simulink model "ContinuosBuck_Offine_Control4"  (R2025a)
settings: Solver=VariableStepAuto  StartTime=0.0  StopTime=SimTime  RelTol=RelativeTolerance
undefined symbols (not defined in the file): C_buck, Iout_buck, kd, ki, kp, L_buck, R, Tsim, Vg, Vout_buck
libraries: slpidlib x1, spsPWMGeneratorDCDCLib x1
settings Model: Creator=Andres  LastModifiedBy=Andres
settings DataIOCC: ReturnWorkspaceOutputs=off  SignalLoggingName=ResultCont

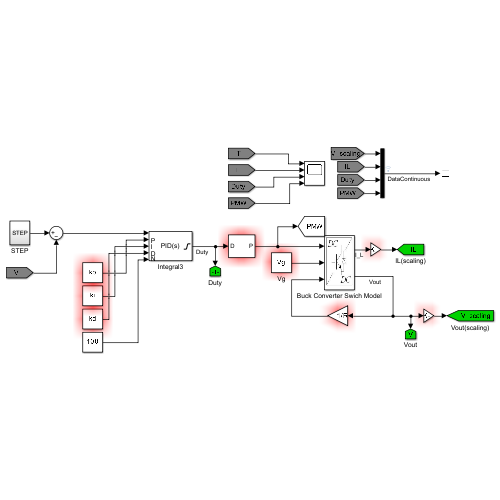
[thumbnail: Simulink's stored preview of the top-level diagram]
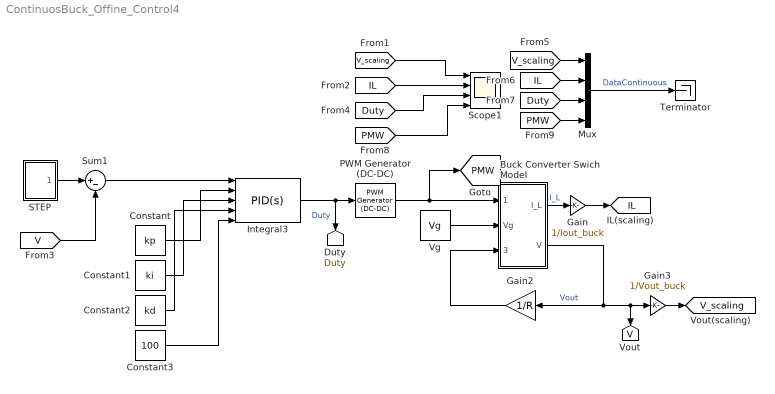
== system ContinuosBuck_Offine_Control4 ==
  Buck Converter Swich Model : Subsystem
      mask Display: image('$imagefile'); % Use "Edit Image" on toolstrip to change.
  Constant : Constant  Value=kp
  Constant1 : Constant  Value=ki
  Constant2 : Constant  Value=kd
  Constant3 : Constant  Value=100
  Gain : Gain  Gain=1/Iout_buck
  Gain2 : Gain  Gain=1/R
  Gain3 : Gain  Gain=1/Vout_buck
  Integral3 : slpidlib/PID Controller  Controller=PID  Form=Parallel  TimeDomain=Continuous-time  UseExternalTs=on  SampleTime=-1  IntegratorMethod=Trapezoidal  FilterMethod=Forward Euler  ControllerParametersSource=external  P=0  I=63.9226  UseKiTs=off  D=0  UseExternalDerivativeSource=off  N=100  UseFilter=on  TunerSelectOption=Transfer Function Based (PID Tuner App)  InitialConditionSource=internal  InitialConditionForIntegrator=0  InitialConditionForFilter=0  DifferentiatorICPrevScaledInput=0  ExternalReset=none  IgnoreLimit=on  TrackingMode=off  Kt=1  LimitOutput=on  SatLimitsSource=internal  UpperSaturationLimit=0.98  LowerSaturationLimit=0  LinearizeAsGain=on  AntiWindupMode=clamping  Kb=1  LimitIntegrator=off  UpperIntegratorSaturationLimit=inf  LowerIntegratorSaturationLimit=-inf  POutMin=[]  POutMax=[]  IOutMin=[]  IOutMax=[]  DOutMin=[]  DOutMax=[]  NOutMin=[]  NOutMax=[]  SumOutMin=[]  SumOutMax=[]  SaturationOutMin=[]  SaturationOutMax=[]  PParamMin=[]  PParamMax=[]  IParamMin=[]  IParamMax=[]  DParamMin=[]  DParamMax=[]  NParamMin=[]  NParamMax=[]  KbParamMin=[]  KbParamMax=[]  KtParamMin=[]  KtParamMax=[]  KbOutMin=[]  KbOutMax=[]  KtOutMin=[]  KtOutMax=[]  IntegratorOutMin=[]  IntegratorOutMax=[]  FilterOutMin=[]  FilterOutMax=[]  SumI1OutMin=[]  SumI1OutMax=[]  SumI2OutMin=[]  SumI2OutMax=[]  SumI3OutMin=[]  SumI3OutMax=[]  SumI4OutMin=[]  SumI4OutMax=[]  SumDOutMin=[]  SumDOutMax=[]  DifferentiatorOutMin=[]  DifferentiatorOutMax=[]  FilterDiffOutCoefMin=[]  FilterDiffOutCoefMax=[]  ReciprocalOutMin=[]  ReciprocalOutMax=[]  SumDenOutMin=[]  SumDenOutMax=[]  SumNumOutMin=[]  SumNumOutMax=[]  DivideOutMin=[]  DivideOutMax=[]  UdiffTsProdOutMin=[]  UdiffTsProdOutMax=[]  NTsProdOutMin=[]  NTsProdOutMax=[]  UintegralTsProdOutMin=[]  UintegralTsProdOutMax=[]  UngainTsProdOutMin=[]  UngainTsProdOutMax=[]  ClampingZeroOutDataTypeStr=Inherit: Inherit via back propagation  ClampingZeroOutMin=[]  ClampingZeroOutMax=[]  FilterDenConstantOutDataTypeStr=Inherit: Inherit via back propagation  FilterDenConstantOutMin=[]  FilterDenConstantOutMax=[]  PCopyOutDataTypeStr=Inherit: Inherit via back propagation  PCopyOutMin=[]  PCopyOutMax=[]  NCopyOutDataTypeStr=Inherit: Inherit via back propagation  NCopyOutMin=[]  NCopyOutMax=[]  IntegratorContinuousStateAttributes=''  IntegratorStateMustResolveToSignalObject=off  IntegratorRTWStateStorageClass=Auto  FilterContinuousStateAttributes=''  FilterStateMustResolveToSignalObject=off  FilterRTWStateStorageClass=Auto  ParallelPVariant=ExternalParameters  IdealPVariant=Disabled  IVariant=ExternalParameters  DVariant=ExternalParameters  IntegratorVariant=Continuous  SatVariant=Enabled  AWVariant=ContClampingParallel  PCopyVariant=Disabled  TRVariant=Disabled  FdbkBlocksVariant=Forward  IdealPFdbkVariant=Disabled  SatFdbkVariant=Disabled  DerivativeFilterVariant=ContFilter  NVariant=ExternalParameters  NCopyVariant=Disabled  FilterICVariant=InternalICsFilter  IntegratorICVariant=InternalICs  ExternalResetVariant=Disabled  TRSumVariant=Passthrough  SumFdbkVariant=Disabled  SumVariant=Sum_PID  TsampFilterVariant=InternalTs  TsampNgainVariant=Passthrough  TsampIntegralVariant=Disabled_SignalSpec  ExternalSaturationOutDataTypeStr=Inherit: Same as second input  DerivativeSourceVariant=ErrorSignal  PreIntVariant=InternalPreInt
  Mux : Mux
  PWM Generator (DC-DC) : spsPWMGeneratorDCDCLib/PWM Generator (DC-DC)  Fsw=f_sw  Ts=0
  STEP : Subsystem
  Scope1 : Scope  NumInputPorts=4
      settings: ActiveDisplayYMinimum=-0.19152108023888853  ActiveDisplayYMaximum=1.7236897221499974  YLabel=Voltage (V)
  Sum1 : Sum  Inputs=|+-
  Terminator : Terminator
  Vg : Constant  Value=Vg  SampleTime=-1
  tag scope: Duty=global, IL=global, PMW=global, V=global, V_scaling=global
  wires:
  Integral3/1 -> [Duty], PWM Generator (DC-DC)/1  "Duty"
  STEP/1(STEP) -> Sum1/1
  [V] -> Sum1/2
  Sum1/1 -> Integral3/1
  Gain2/1 -> Buck Converter Swich Model/3(I_load)
  Buck Converter Swich Model/1(I_L) -> Gain/1  "I_L"
  Buck Converter Swich Model/2(V) -> Gain2/1, [V], Gain3/1  "Vout"
  PWM Generator (DC-DC)/1 -> [PMW], Buck Converter Swich Model/1(PWM)
  Vg/1 -> Buck Converter Swich Model/2(Vg)
  Mux/1 -> Terminator/1  "DataContinuous"
  Gain3/1 -> [V_scaling]
  Gain/1 -> [IL]
  [V_scaling] -> Scope1/1
  [IL] -> Scope1/2
  [Duty] -> Scope1/3
  [V_scaling] -> Mux/1
  [IL] -> Mux/2
  [Duty] -> Mux/3
  [PMW] -> Scope1/4
  [PMW] -> Mux/4
  Constant/1 -> Integral3/2
  Constant1/1 -> Integral3/3
  Constant2/1 -> Integral3/4
  Constant3/1 -> Integral3/5

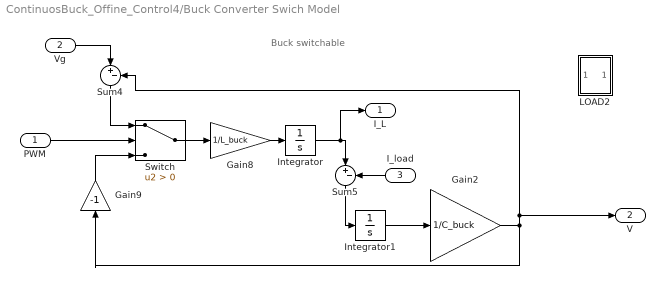
== system ContinuosBuck_Offine_Control4/Buck Converter Swich Model ==
  note: Buck switchable
  PWM : Inport
  Vg : Inport  Port=2
  I_load : Inport  Port=3
  Gain2 : Gain  Gain=1/C_buck
  Gain8 : Gain  Gain=1/L_buck
  Gain9 : Gain  Gain=-1
  Integrator : Integrator  LimitOutput=on  LowerSaturationLimit=0
  Integrator1 : Integrator
  LOAD2 : Subsystem
  Sum4 : Sum  Inputs=|+-
  Sum5 : Sum  Inputs=|+-
  Switch : Switch  Criteria=u2 > Threshold  SaturateOnIntegerOverflow=off  InputSameDT=off
  I_L : Outport
  V : Outport  Port=2
  wires:
  Gain9/1 -> Switch/3
  Switch/1 -> Gain8/1
  Sum4/1 -> Switch/1
  Gain8/1 -> Integrator/1
  Sum5/1 -> Integrator1/1
  Integrator/1 -> I_L/1, Sum5/1
  Vg/1 -> Sum4/1
  I_load/1 -> Sum5/2
  PWM/1 -> Switch/2
  Gain2/1 -> Gain9/1, V/1, Sum4/2
  Integrator1/1 -> Gain2/1

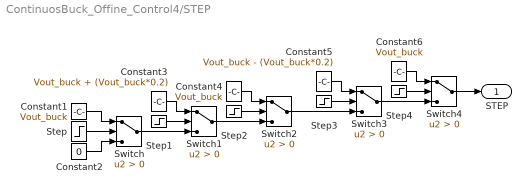
== system ContinuosBuck_Offine_Control4/STEP ==
  Constant1 : Constant  Value=Vout_buck  SampleTime=-1
  Constant2 : Constant  Value=0  SampleTime=-1
  Constant3 : Constant  Value=Vout_buck + (Vout_buck*0.2)  SampleTime=-1
  Constant4 : Constant  Value=Vout_buck  SampleTime=-1
  Constant5 : Constant  Value=Vout_buck - (Vout_buck*0.2)  SampleTime=-1
  Constant6 : Constant  Value=Vout_buck  SampleTime=-1
  Step : Step  Time=0.01
  Step1 : Step  Time=0.02
  Step2 : Step  Time=0.03
  Step3 : Step  Time=0.04
  Step4 : Step  Time=0.05
  Switch{,1..4} (5 alike) : Switch  Criteria=u2 > Threshold  SaturateOnIntegerOverflow=off  InputSameDT=off
  STEP : Outport
  wires:
  Step/1 -> Switch/2
  Constant3/1 -> Switch1/1
  Constant1/1 -> Switch/1
  Switch/1 -> Switch1/3
  Step1/1 -> Switch1/2
  Constant2/1 -> Switch/3
  Switch1/1 -> Switch2/3
  Step2/1 -> Switch2/2
  Constant4/1 -> Switch2/1
  Constant5/1 -> Switch3/1
  Switch2/1 -> Switch3/3
  Step3/1 -> Switch3/2
  Constant6/1 -> Switch4/1
  Switch3/1 -> Switch4/3
  Step4/1 -> Switch4/2
  Switch4/1 -> STEP/1

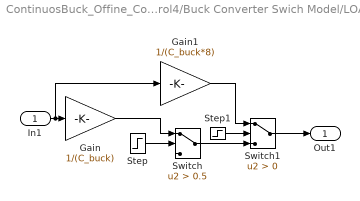
== system ContinuosBuck_Offine_Control4/Buck Converter Swich Model/LOAD2 ==
  In1 : Inport
  Gain : Gain  Gain=1/(C_buck)
  Gain1 : Gain  Gain=1/(C_buck*8)
  Step : Step  Time=0  SampleTime=Tsim
  Step1 : Step  Time=0.07  SampleTime=Tsim
  Switch : Switch  Criteria=u2 > Threshold  Threshold=0.5  SaturateOnIntegerOverflow=off  InputSameDT=off
  Switch1 : Switch  Criteria=u2 > Threshold  SaturateOnIntegerOverflow=off  InputSameDT=off
  Out1 : Outport
  wires:
  Gain1/1 -> Switch1/1
  Step/1 -> Switch/2
  Switch/1 -> Switch1/3
  Step1/1 -> Switch1/2
  Switch1/1 -> Out1/1
  In1/1 -> Gain/1, Gain1/1
  Gain/1 -> Switch/1
